simulink model "ZigBee"  (R2017a)
settings: Solver=ode23t  StartTime=0.0  StopTime=inf  FixedStep=SampTime  RelTol=1e-3  EnableMultiTasking=on
PreLoadFcn:
  | %Data Rates
  | BitRate=(250)*1e3;
  | ChipRate=2e6;
  | SymRate=ChipRate/2;
  | OS=32; %Pulse shaping filter oversampling
  | SampRate=OS*SymRate;
  | SampTime=1/SampRate;
  | 
  | %BER overhead
  | RX_ChipDelay=6;
  | 
  | %Signal Specs
  | Pin=-40;
  | fc_RF=2450e6;
  | 
  | %Interference Specs
  | fc_BL=2500e6;
  | INT_CHRT=3.846e6; %chip rate
  | INT_SPS=32; %up-sampling rate
  | INT_RO=0.22; %pulse shaping filter param
  | INT_PWR=0; %passband Power
  | 
  | %Receiver Design + Impairements
  | Gain_LNA=20;
  | IIP2_LNA=inf;
  | IIP3_LNA=inf;
  | NF_LNA=2.5;
  | 
  | Gain_MIX=-5;
  | IIP2_MIX=60;
  | IIP3_MIX=inf;
  | NF_MIX=9;
  | 
  | Gain_VGA=44-15;
  | IIP2_VGA=inf;
  | IIP3_VGA=inf;
  | NF_VGA=12;
  | 
  | ADC_FSP=0;
  | ADC_RES=10;
  | 
  | FLICKER_KERN=2^11;
  | FLICKER_CORNER=10e3;
  | FLICKER_PSD_FLOOR=-124;
  | 
  | PLL_NOISE=[-80 -80 -80 -80 -85 -95];
  | PLL_FREQ=[0.01 0.1 1 2 3 7]*1e6;
  | PLL_KERN=2000;
InitFcn:
  | x=linspace(0,1,OS);
  | weights=sin(pi*x);
undefined symbols (not defined in the file or in its folder): dfilt, Frame, Fs, gcbh, rcfiltgaincompat
libraries: simrfV2elements x9, simulink x5, simrfV2util1 x5, dspstat3 x4, commdigbbndpm3 x3, dspmathops x3, dspobslib x3, simrfV2_lib x3, dspmlti4 x2, dsparch4 x2, commutil2 x1, commrflib2 x1
settings Model: Creator=The MathWorks Inc.  LastModifiedBy=gzucchel
settings DataIOCC: LimitDataPoints=on  SaveFormat=Array  SignalLoggingSaveFormat=ModelDataLogs  SaveOutput=off  SignalLogging=off  DSMLogging=off  SaveTime=off
settings OptimizationCC: ExpressionDepthLimit=2147483647  LifeSpan=inf
settings DebuggingCC: ConsistencyChecking=warning  UnderspecifiedInitializationDetection=Classic  MergeDetectMultiDrivingBlocksExec=none  TimeAdjustmentMsg=warning  MaxConsecutiveZCsMsg=warning  SolverPrmCheckMsg=warning  FcnCallInpInsideContextMsg=warning  ModelReferenceExtraNoncontSigs=warning  StateNameClashWarn=warning  SimStateOlderReleaseMsg=warning  SFUnexpectedBacktrackingDiag=warning  SFNoUnconditionalDefaultTransitionDiag=warning  SFExecutionAtInitializationDiag=none
settings HardwareCC: ProdBitPerPointer=32  ProdBitPerSizeT=32  ProdBitPerPtrDiffT=32  ProdLargestAtomicFloat=None  ProdIntDivRoundTo=Undefined  ProdEndianess=Unspecified  ProdWordSize=32  ProdHWDeviceType=32-bit Generic
settings ModelReferenceCC: PropagateSignalLabelsOutOfModel=off
settings GRTTargetCC: TargetLangStandard=C89/C90 (ANSI)  GeneratePreprocessorConditionals=Disable all  CombineOutputUpdateFcns=off  GRTInterface=on
settings ConfigComp: CovMetricSettings=dw  CovHtmlReporting=on  CovSaveCumulativeToWorkspaceVar=on  CovSaveSingleToWorkspaceVar=on  CovExternalEMLEnable=off  CovSFcnEnable=off
settings ConfigurationSet: Description=SimMechanics 2G

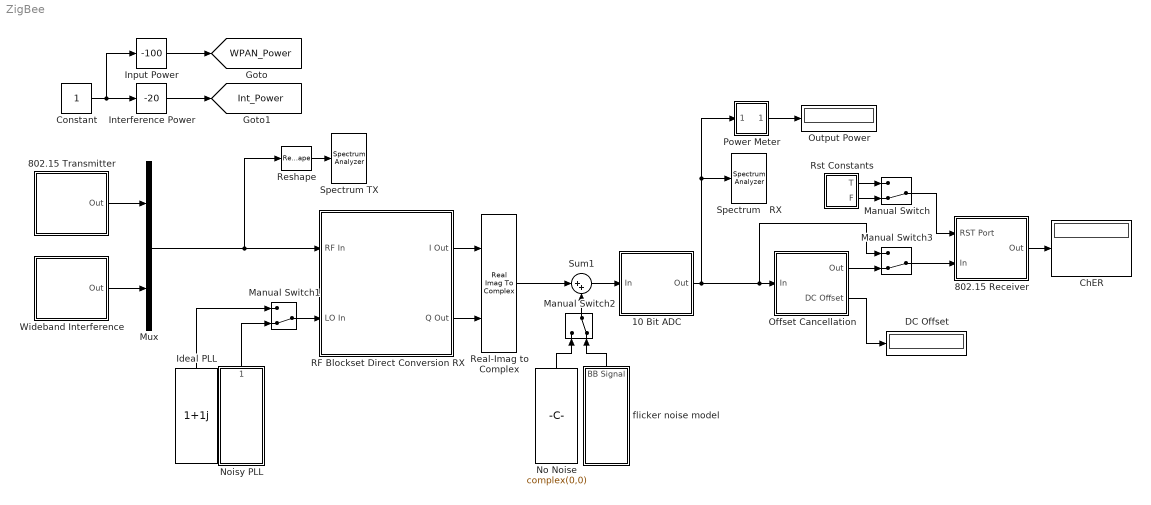
== system ZigBee ==
  10 Bit ADC : Subsystem  mask{FS_P_dBm=0, Rnorm=1, N=10, Sample_Rate=0.0}
      mask prompts: FS_P_dBm "Full Scale Power"; Rnorm "Normalization Resistance"; Sample_Rate "Sample Rate (-1 for inherited)"
      mask init:
      | %LSB=FS_V/(2^(N-1));
      | %MAX=FS_V-LSB;
      | %MIN=-FS_V+LSB;
      | LSB=sqrt(2*Rnorm)*sqrt(1e-3)*sqrt(10^(FS_P_dBm/10))/(2^(N-1));
      | MAXp=sqrt(2*Rnorm)*sqrt(1e-3)*sqrt(10^(FS_P_dBm/10))-LSB;
      | MINp=-sqrt(2*Rnorm)*sqrt(1e-3)*sqrt(10^(FS_P_dBm/10))+LSB;
  802.15 Receiver : Subsystem
  802.15 Transmitter : Subsystem
  ChER : Display
  Constant : Constant
  DC Offset : Display
  Ideal PLL : Constant  Value=1+1j  VectorParams1D=off  SampleTime=1/SampRate  FramePeriod=Frame/Fs
  "Input Power " : simulink/Math Operations/Slider Gain  gain=-100  low=-120  high=-30
  "Interference Power " : simulink/Math Operations/Slider Gain  gain=-20  low=-200  high=0
  Manual Switch{,1..3} (4 alike) : ManualSwitch  CurrentSetting=0
  Mux : Mux  Inputs=2
  No Noise : Constant  Value=complex(0,0)  VectorParams1D=off  SampleTime=1/SampRate  FramePeriod=Frame/Fs
  Noisy PLL : Subsystem  mask{Level_dB=PLL_NOISE, Freq=PLL_FREQ, Fs=SampRate, Npts=PLL_KERN, seed=159775318}
      mask prompts: Level_dB "Noise Level Vector in dBc/Hz"; Freq "Frequency Vector in Hz"; Fs "Sampling Rate in Hz"; Npts "FIR Filter Kernel Length"; seed "Noise Gen Seed"
  Offset Cancellation : Subsystem
  Output Power : Display
  Power Meter : Subsystem  mask{R=1, PB=off, buffer_sz=32*32}
      mask prompts: R "Resistance"; PB "Passband Power (Divide by 2)"; buffer_sz "Buffer Size"
  RF Blockset Direct Conversion RX : Subsystem
  Real-Imag to Complex : RealImagToComplex
  Reshape : Reshape  OutputDimensionality=Row vector (2-D)
  Rst Constants : Subsystem
  Spectrum   RX : SpectrumAnalyzer
  Spectrum TX : SpectrumAnalyzer
  Sum1 : Sum  Inputs=|++
  Wideband Interference : Subsystem
  flicker noise model : Subsystem
  tag scope: Int_Power=global, WPAN_Power=global
  wires:
  802.15 Receiver/1(Out) -> ChER/1
  802.15 Transmitter/1(Out) -> Mux/1
  RF Blockset Direct Conversion RX/1(I Out) -> Real-Imag to Complex/1
  RF Blockset Direct Conversion RX/2(Q Out) -> Real-Imag to Complex/2
  Sum1/1 -> 10 Bit ADC/1(In)
  "Interference Power "/1 -> [Int_Power]
  "Input Power "/1 -> [WPAN_Power]
  10 Bit ADC/1(Out) -> Manual Switch3/1, Offset Cancellation/1(In), Power Meter/1(In), Spectrum   RX/1
  Mux/1 -> RF Blockset Direct Conversion RX/1(RF In), Reshape/1
  Constant/1 -> "Input Power "/1, "Interference Power "/1
  Real-Imag to Complex/1 -> Sum1/1
  Rst Constants/1(T) -> Manual Switch/1
  Rst Constants/2(F) -> Manual Switch/2
  Manual Switch/1 -> 802.15 Receiver/1(RST Port)
  Wideband Interference/1(Out) -> Mux/2
  Manual Switch1/1 -> RF Blockset Direct Conversion RX/2(LO In)
  Noisy PLL/1(PLL Output) -> Manual Switch1/2
  Ideal PLL/1 -> Manual Switch1/1
  Manual Switch2/1 -> Sum1/2
  flicker noise model/1(BB Signal) -> Manual Switch2/2
  No Noise/1 -> Manual Switch2/1
  Power Meter/1(Power) -> Output Power/1
  Offset Cancellation/2(DC Offset) -> DC Offset/1
  Offset Cancellation/1(Out) -> Manual Switch3/2
  Manual Switch3/1 -> 802.15 Receiver/2(In)
  Reshape/1 -> Spectrum TX/1

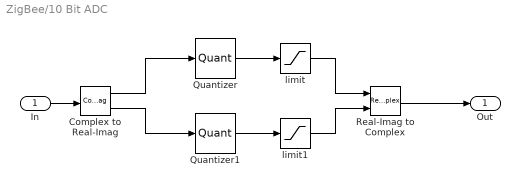
== system ZigBee/10 Bit ADC ==
  In : Inport
  Complex to Real-Imag : ComplexToRealImag
  Quantizer : Quantizer  QuantizationInterval=LSB
  Quantizer1 : Quantizer  QuantizationInterval=LSB
  Real-Imag to Complex : RealImagToComplex
  limit : Saturate  UpperLimit=MAXp  LowerLimit=MINp
  limit1 : Saturate  UpperLimit=MAXp  LowerLimit=MINp
  Out : Outport
  wires:
  Quantizer/1 -> limit/1
  In/1 -> Complex to Real-Imag/1
  Complex to Real-Imag/1 -> Quantizer/1
  Quantizer1/1 -> limit1/1
  Complex to Real-Imag/2 -> Quantizer1/1
  limit/1 -> Real-Imag to Complex/1
  limit1/1 -> Real-Imag to Complex/2
  Real-Imag to Complex/1 -> Out/1

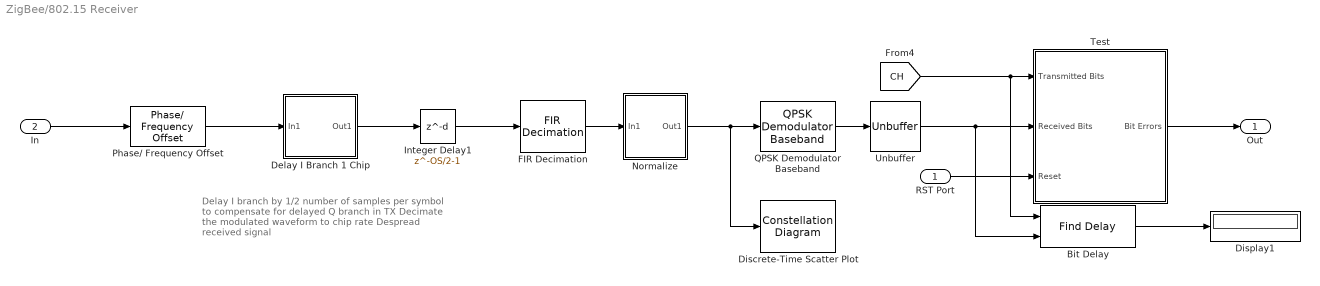
== system ZigBee/802.15 Receiver ==
  note: Delay I branch by 1/2 number of samples per
      | symbol to compensate for delayed Q branch in TX
      |
      | Decimate the modulated waveform to chip rate
      |
      | Despread received signal
  RST Port : Inport
  In : Inport  Port=2
  Bit Delay : commutil2/Find Delay  corrLength=20  chgSigOP=off  stopUpdate=off  numConstDelay=3
      settings: SourceProductName=Communications System Toolbox  SourceProductBaseCode=CM
  Delay I Branch 1 Chip : Subsystem
  Discrete-Time Scatter Plot : ConstellationDiagram  Tag=ScatterPlot
  Display1 : Display
  FIR Decimation : dspmlti4/FIR Decimation  FilterSource=Dialog parameters  h=fliplr(conj(weights))  D=OS  filtStruct=Direct form  FilterObject=Hm_firdecim  InputProcessing=Columns as channels (frame based)  framing=Allow multirate processing  inputOffset=0  outputBufInitCond=0  roundingMode=Floor  overflowMode=off  firstCoeffDataTypeStr=Inherit: Same word length as input  firstCoeffMin=[]  firstCoeffMax=[]  firstCoeffLastDataTypeStr=Inherit: Same word length as input  outputDataTypeStr=Inherit: Same as accumulator  outputMin=[]  outputMax=[]  outputLastDataTypeStr=Inherit: Same as accumulator
  Integer Delay1 : Delay  DelayLength=OS/2-1
  Normalize : Subsystem
  Phase/ Frequency Offset : commrflib2/Phase// Frequency Offset  phaseOffset=58  freqPort=off  freqOffset=0
      settings: SourceProductName=Communications System Toolbox
  QPSK Demodulator Baseband : commdigbbndpm3/QPSK Demodulator Baseband  OutType=Bit  DecType=Hard decision  VarSource=Dialog  Variance=1  Dec=Gray  Ph=pi/4  outDtype1=Inherit via internal rule  outDtype2=Inherit via internal rule  derotateFactorWordLen=16  derotateFactorDataTypeStr=Inherit: Same word length as input  derotateFactorLastDataTypeStr=Inherit: Same word length as input
  Test : Subsystem
  Unbuffer : Unbuffer
  Out : Outport
  wires:
  Test/1(Bit Errors) -> Out/1
  Bit Delay/1 -> Display1/1
  Delay I Branch 1 Chip/1(Out1) -> Integer Delay1/1
  In/1 -> Phase/ Frequency Offset/1
  QPSK Demodulator Baseband/1 -> Unbuffer/1
  Unbuffer/1 -> Test/2(Received Bits), Bit Delay/2
  Integer Delay1/1 -> FIR Decimation/1
  FIR Decimation/1 -> Normalize/1(In1)
  [CH] -> Test/1(Transmitted Bits), Bit Delay/1
  Phase/ Frequency Offset/1 -> Delay I Branch 1 Chip/1(In1)
  Normalize/1(Out1) -> QPSK Demodulator Baseband/1, Discrete-Time Scatter Plot/1
  RST Port/1 -> Test/3(Reset)

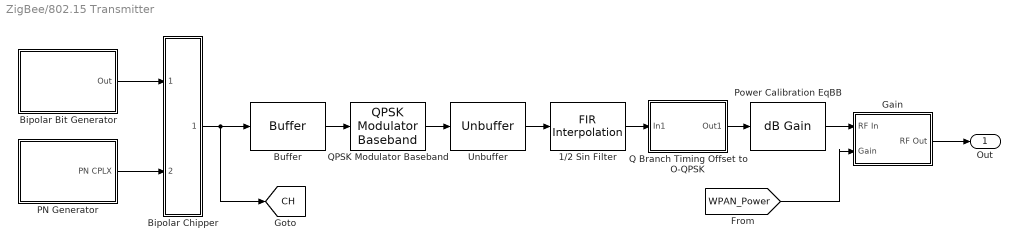
== system ZigBee/802.15 Transmitter ==
  1/2 Sin Filter : dspmlti4/FIR Interpolation  FilterSource=Dialog parameters  h=weights  L=OS  FilterObject=Hm_firinterp  framing=Allow multirate processing  outputBufInitCond=0  roundingMode=Floor  overflowMode=off  firstCoeffDataTypeStr=Inherit: Same word length as input  firstCoeffMin=[]  firstCoeffMax=[]  firstCoeffLastDataTypeStr=Inherit: Same word length as input  outputDataTypeStr=Inherit: Same as accumulator  outputMin=[]  outputMax=[]  outputLastDataTypeStr=Inherit: Same as accumulator
      settings: SourceProductName=DSP System Toolbox
  Bipolar Chipper : Subsystem
  Bipolar Bit Generator : Subsystem
  Buffer : Buffer  N=2
  Gain : Subsystem
  PN Generator : Subsystem
  Power Calibration EqBB : dspmathops/dB Gain  dB=-26.8  intype=Amplitude
      settings: SourceProductName=DSP System Toolbox  SourceProductBaseCode=DS
  Q Branch Timing Offset to O-QPSK : Subsystem
  QPSK Modulator Baseband : commdigbbndpm3/QPSK Modulator Baseband  InType=Bit  Enc=Gray  Ph=pi/4  outDtype=double  outWordLen=16  outUDDataType=sfix(16)  outFracLenMode=Best precision  outFracLen=15  outDataTypeStr=double  outLastDataTypeStr=double
  Unbuffer : Unbuffer
  Out : Outport
  tag scope: CH=global
  wires:
  Power Calibration EqBB/1 -> Gain/1(RF In)
  Gain/1(RF Out) -> Out/1
  Q Branch Timing Offset to O-QPSK/1(Out1) -> Power Calibration EqBB/1
  [WPAN_Power] -> Gain/2(Gain)
  Unbuffer/1 -> 1/2 Sin Filter/1
  Buffer/1 -> QPSK Modulator Baseband/1
  Bipolar Chipper/1(Out) -> [CH], Buffer/1
  Bipolar Bit Generator/1(Out) -> Bipolar Chipper/1(In1)
  PN Generator/1(PN CPLX) -> Bipolar Chipper/2(In2)
  1/2 Sin Filter/1 -> Q Branch Timing Offset to O-QPSK/1(In1)
  QPSK Modulator Baseband/1 -> Unbuffer/1

== system ZigBee/Noisy PLL ==
  Constant : Constant  VectorParams1D=off  SampleTime=1/Fs  FramePeriod=Frame/Fs
  Phase Noise1 : Subsystem  Description=|  mask{Level_dB=Level_dB, Freq=Freq, Fs=Fs, Npts=Npts, seed=seed, Verify=off}
      | User defined phase noise block.
      | Dick Benson, May 2007
      mask prompts: Level_dB "Noise Level Vector in dBc/Hz"; Freq "Frequency Vector in Hz"; Fs "Sampling Rate in Hz"; Npts "FIR Filter Kernel Length (power of 2)"; seed "Noise Gen. Seed"; Verify "Verify Noise Shape Attained"
      mask init:
      | noise_filt=phaseNoise(Npts, Freq, Level_dB, Fs,Verify);
      mask Display: disp('Prototype\nPhase Noise\nBlock')
  Real-Imag to Complex : RealImagToComplex  Input=Real
  PLL Output : Outport
  wires:
  Phase Noise1/1(Out1) -> PLL Output/1
  Real-Imag to Complex/1 -> Phase Noise1/1(In1)
  Constant/1 -> Real-Imag to Complex/1

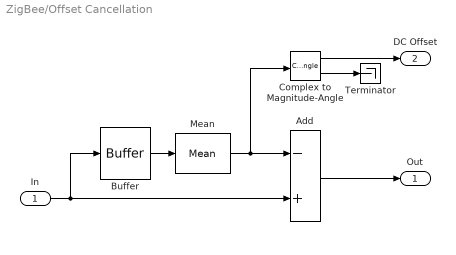
== system ZigBee/Offset Cancellation ==
  In : Inport
  Add : Sum  Inputs=-+
  Buffer : Buffer  N=OS*50  V=OS*25
  Complex to Magnitude-Angle : ComplexToMagnitudeAngle
  Mean : dspstat3/Mean  run=off  reset_popup=None  directionMode=Entire input  dimension=1  roiEnable=off  roiType=Rectangles  roiPortion=Entire ROI  roiOutput=Individual statistics for each ROI  roiFlag=off  outputDataTypeStr=Inherit: Same as accumulator  outputLastDataTypeStr=Inherit: Same as accumulator  outputMin=[]  outputMax=[]  roundingMode=Floor  overflowMode=off
  Terminator : Terminator
  Out : Outport
  DC Offset : Outport  Port=2
  wires:
  Add/1 -> Out/1
  Mean/1 -> Add/1, Complex to Magnitude-Angle/1
  In/1 -> Add/2, Buffer/1
  Buffer/1 -> Mean/1
  Complex to Magnitude-Angle/1 -> DC Offset/1
  Complex to Magnitude-Angle/2 -> Terminator/1

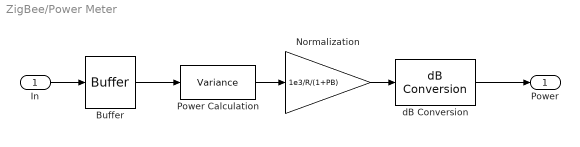
== system ZigBee/Power Meter ==
  In : Inport
  Buffer : Buffer  N=buffer_sz
  Normalization : Gain  Gain=1e3/R/(1+PB)
  Power Calculation : dspstat3/Variance  run=off  reset_popup=None  InputProcessing=Columns as channels (frame based)  directionMode=Each column  dimension=1  roiEnable=off  roiType=Rectangles  roiPortion=Entire ROI  roiOutput=Individual statistics for each ROI  roiFlag=off  roundingMode=Floor  overflowMode=off
      settings: SourceProductName=DSP System Toolbox
  dB Conversion : dspmathops/dB Conversion  dBtype=dB  intype=Power  R=1  fuzz=on
      settings: SourceProductName=DSP System Toolbox
  Power : Outport
  wires:
  Power Calculation/1 -> Normalization/1
  Normalization/1 -> dB Conversion/1
  In/1 -> Buffer/1
  Buffer/1 -> Power Calculation/1
  dB Conversion/1 -> Power/1

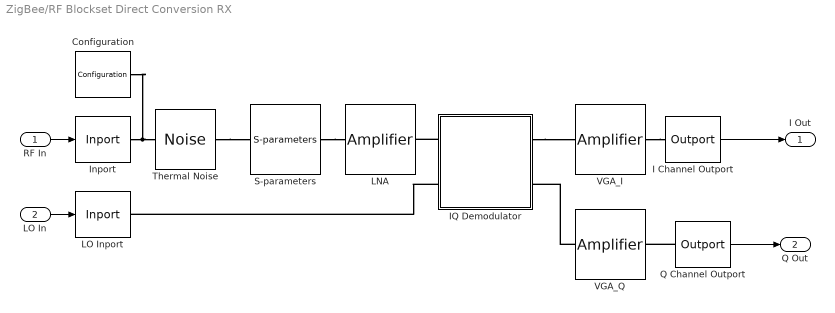
== system ZigBee/RF Blockset Direct Conversion RX ==
  RF In : Inport
  LO In : Inport  Port=2
  Configuration : simrfV2util1/Configuration  AutoFreq=off  Tones="[2.45         2.5] GHz"  Harmonics=[1 3]  NormalizeCarrierPower=on  SolverType=Auto  UseCCode=on  StepSize=SampTime s  AddNoise=on  defaultRNG=on  Seed=0  Temperature=290 K  SolverDelFlag=0  AbsTol=1e-6  RelTol=1e-3  MaxIter=10  ErrorEstimationType=2-norm over all variables
      settings: SourceProductName=RF Blockset  SourceProductBaseCode=RB
  I Channel Outport : simrfV2util1/Outport  SensorType=Power  OutputFormat=Real Passband  CarrierFreq=0 Hz  ZL=100  InternalGrounding=on  StepSize=-1 s  AutoStep=off
      settings: SourceProductName=RF Blockset  SourceProductBaseCode=RB
  IQ Demodulator : Subsystem  DialogController=simrfV2DDGCreate  mask(IQ Demodulator){classname=iqdemod, Source_linear_gain=Available power gain, linear_gain=Gain_MIX, linear_gain_unit=dB, Zin=50, Zout=50, Source_Poly=Even and odd order, Poly_Coeffs=[0 1], IPType=Input, IP2=IIP2_MIX, IP2_unit=dBm, IP3=IIP3_MIX, IP3_unit=dBm, P1dB=inf, P1dB_unit=dBm, Psat=inf, Psat_unit=dBm, Gcomp=inf, Gcomp_unit=dBm, NF=NF_MIX, InternalGrounding=on, LOFreq=0, LOFreq_unit=Hz, GainMismatch=0, GainMismatch_unit=dB, PhaseMismatch=0, PhaseMismatch_unit=deg, Isolation=50, Isolation_unit=dB}
      mask prompts: classname "Class name:"; Source_linear_gain "Gain option:"; linear_gain "Linear gain:"; linear_gain_unit "Linear gain unit:"; Zin "Input impedance:"; Zout "Output impedance:"; Source_Poly "Source of cubic polynomial:"; Poly_Coeffs "Polynomial coefficients:"; IPType "Intercept points at:"; IP2_unit "IP2 unit:"; IP3_unit "IP3 unit:"; P1dB_unit "P1dB unit:"; Psat_unit "Psat unit:"; Gcomp_unit "Gcomp unit:"; NF "Noise figure (dB):"; InternalGrounding "Ground and hide negative terminals."; LOFreq "Local oscillator frequency"; LOFreq_unit "Local oscillator frequency unit:"; GainMismatch "I/Q gain mismatch"; GainMismatch_unit "I/Q gain mismatch unit:"; PhaseMismatch "I/Q phase mismatch:"; PhaseMismatch_unit "I/Q phase mismatch unit:"; Isolation "LO to RF isolation:"; Isolation_unit "LO to RF isolation unit:"
      mask help: Model an IQ demodulator
      mask init:
      | iqDemodMaskParams = simrfV2iqdemod(gcb, 'simrfInit'); % iqDemodMaskParams contains parameters that are verified and converted to standard units
      | 
      | % Assignment to internal block parameters is done only at compile time
      | if regexpi(get_param(bdroot(gcb), 'SimulationStatus'), ...
      |         '^(updating|initializing)$')
      |     % iqDemodParams contains parameters used by internal blocks
      |     iqDemodParams = simrfV2_iqdemod_params(iqDemodMaskParams);
      | end
      mask Help: eval('simrfV2_help(gcbh)')
      mask TypeOptions Source_linear_gain: Available power gain | Open circuit voltage gain | Polynomial coefficients
      mask TypeOptions linear_gain_unit: dB | None
      mask TypeOptions Source_Poly: Even and odd order | Odd order
      mask TypeOptions IPType: Output | Input
      mask TypeOptions IP2_unit: W | mW | dBW | dBm
      mask TypeOptions IP3_unit: W | mW | dBW | dBm
      mask TypeOptions P1dB_unit: W | mW | dBW | dBm
      mask TypeOptions Psat_unit: W | mW | dBW | dBm
      mask TypeOptions Gcomp_unit: W | mW | dBW | dBm
      mask TypeOptions LOFreq_unit: Hz | kHz | MHz | GHz
      mask TypeOptions GainMismatch_unit: dB | None
      mask TypeOptions PhaseMismatch_unit: rad | deg
      mask TypeOptions Isolation_unit: dB | None
      mask Display:
      | simrfV2icon_iqdemod
      | text(0.5+0.15,0.5+0.075,'LO')
      | port_label('LConn', 1,'In')
      | port_label('RConn', 1,'I')
      | port_label('RConn', 2,'Q')
  Inport : simrfV2util1/Inport  SimulinkInputSignalType=Power  CarrierFreq=[fc_RF,fc_BL] Hz  ZS=50  InternalGrounding=on
      settings: SourceProductName=RF Blockset  SourceProductBaseCode=RB
  LNA : simrfV2elements/Amplifier  classname=amplifier  DataSource=Data file  File=unitygain.s2p  Paramtype=S-parameters  Sparam=[0 0;1 0]  SparamFreq=1e9 Hz  SparamZ0=50  Residues=0  Poles=0  DF={0 0; 1 0}  Source_linear_gain=Available power gain  linear_gain=Gain_LNA dB  Zin=50  Zout=50  Source_Poly=Even and odd order  Poly_Coeffs=[0 1]  IPType=Input  IP2=IIP2_LNA dBm  IP3=IIP3_LNA dBm  P1dB=inf dBm  Psat=inf dBm  Gcomp=inf dBm  NF=NF_LNA+1  InternalGrounding=on  SourceFreq=Extracted from data source  PlotFreq=0 Hz  PlotType=X-Y plane  YParam1=S11  YFormat1=Magnitude (decibels)  YParam2=None  YFormat2=Magnitude (decibels)  YOption=Linear  XOption=Linear  SparamRepresentation=Time domain (rationalfit)  FitTol=-40  FitOpt=Fit individually  AutoImpulseLength=off  ImpulseLength=0 s
      settings: SourceProductName=RF Blockset  SourceProductBaseCode=RB
  LO Inport : simrfV2util1/Inport  SimulinkInputSignalType=Ideal voltage  CarrierFreq=fc_RF Hz  ZS=0  InternalGrounding=on
      settings: SourceProductName=RF Blockset  SourceProductBaseCode=RB
  Q Channel Outport : simrfV2util1/Outport  SensorType=Power  OutputFormat=Real Passband  CarrierFreq=0 Hz  ZL=100  InternalGrounding=on  StepSize=-1 s  AutoStep=off
      settings: SourceProductName=RF Blockset  SourceProductBaseCode=RB
  S-parameters : simrfV2elements/S-parameters  classname=sparam_element  DataSource=Data file  File=SAW_Filter_Data.s2p  Paramtype=S-parameters  Sparam=[0 0;1 0]  SparamFreq=1e9 Hz  SparamZ0=50  Residues=0  Poles=0  DF={0 0; 1 0}  FitOpt=Share all poles  FitTol=-40  SourceFreq=Extracted from data source  PlotFreq=1 Hz  PlotType=X-Y plane  YParam1=S21  YFormat1=Magnitude (decibels)  YParam2=None  YFormat2=Magnitude (decibels)  YOption=Linear  XOption=Linear  AddNoise=off  InternalGrounding=on  SparamRepresentation=Time domain (rationalfit)  AutoImpulseLength=off  ImpulseLength=0 s
      settings: SourceProductName=RF Blockset  SourceProductBaseCode=RB
  Thermal Noise : simrfV2sources1/Noise  SimulinkInputSignalType=Ideal voltage  NoiseType=White  NoisePSD=4*1.381e-23*290*50  CarrierFreq=fc_RF Hz  InternalGrounding=off
      settings: SourceProductName=RF Blockset  SourceProductBaseCode=RB
  VGA_I : simrfV2elements/Amplifier  classname=amplifier  DataSource=Data file  File=unitygain.s2p  Paramtype=S-parameters  Sparam=[0 0;1 0]  SparamFreq=1e9 Hz  SparamZ0=50  Residues=0  Poles=0  DF={0 0; 1 0}  Source_linear_gain=Available power gain  linear_gain=Gain_VGA dB  Zin=100  Zout=100  Source_Poly=Even and odd order  Poly_Coeffs=[0 1]  IPType=Input  IP2=IIP2_VGA dBm  IP3=IIP3_VGA dBm  P1dB=inf dBm  Psat=inf dBm  Gcomp=inf dBm  NF=NF_VGA  InternalGrounding=on  SourceFreq=Extracted from data source  PlotFreq=0 Hz  PlotType=X-Y plane  YParam1=S11  YFormat1=Magnitude (decibels)  YParam2=None  YFormat2=Magnitude (decibels)  YOption=Linear  XOption=Linear  SparamRepresentation=Time domain (rationalfit)  FitTol=-40  FitOpt=Fit individually  AutoImpulseLength=off  ImpulseLength=0 s
      settings: SourceProductName=RF Blockset  SourceProductBaseCode=RB
  VGA_Q : simrfV2elements/Amplifier  classname=amplifier  DataSource=Data file  File=unitygain.s2p  Paramtype=S-parameters  Sparam=[0 0;1 0]  SparamFreq=1e9 Hz  SparamZ0=50  Residues=0  Poles=0  DF={0 0; 1 0}  Source_linear_gain=Available power gain  linear_gain=Gain_VGA dB  Zin=100  Zout=100  Source_Poly=Even and odd order  Poly_Coeffs=[0 1]  IPType=Input  IP2=IIP2_VGA dBm  IP3=IIP3_VGA dBm  P1dB=inf dBm  Psat=inf dBm  Gcomp=inf dBm  NF=NF_VGA  InternalGrounding=on  SourceFreq=Extracted from data source  PlotFreq=0 Hz  PlotType=X-Y plane  YParam1=S11  YFormat1=Magnitude (decibels)  YParam2=None  YFormat2=Magnitude (decibels)  YOption=Linear  XOption=Linear  SparamRepresentation=Time domain (rationalfit)  FitTol=-40  FitOpt=Fit individually  AutoImpulseLength=off  ImpulseLength=0 s
      settings: SourceProductName=RF Blockset  SourceProductBaseCode=RB
  I Out : Outport
  Q Out : Outport  Port=2
  wires:
  LO In/1 -> LO Inport/1
  RF In/1 -> Inport/1
  Q Channel Outport/1 -> Q Out/1
  I Channel Outport/1 -> I Out/1
  connections:
  VGA_I/RConn1 -- I Channel Outport/LConn1
  Q Channel Outport/LConn1 -- VGA_Q/RConn1
  VGA_Q/LConn1 -- IQ Demodulator/RConn2
  IQ Demodulator/RConn1 -- VGA_I/LConn1
  Inport/RConn1 -- Configuration/LConn1 -- Thermal Noise/RConn1
  S-parameters/RConn1 -- LNA/LConn1
  Thermal Noise/LConn1 -- S-parameters/LConn1
  IQ Demodulator/LConn1 -- LNA/RConn1
  IQ Demodulator/LConn2 -- LO Inport/RConn1

== system ZigBee/Rst Constants ==
  Constant : Constant
  Constant1 : Constant  Value=0
  T : Outport
  F : Outport  Port=2
  wires:
  Constant/1 -> T/1
  Constant1/1 -> F/1

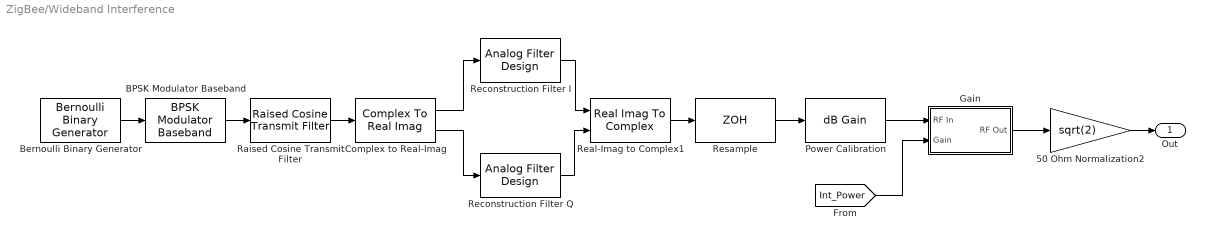
== system ZigBee/Wideband Interference ==
  50 Ohm Normalization2 : Gain  Gain=sqrt(2)
  BPSK Modulator Baseband : commdigbbndpm3/BPSK Modulator Baseband  Ph=0  outDtype=double  outWordLen=16  outUDDataType=sfix(16)  outFracLenMode=Best precision  outFracLen=15  outDataTypeStr=double  outLastDataTypeStr=double
  Bernoulli Binary Generator : commrandsrc2/Bernoulli Binary Generator  P=0.5  seed=61  Ts=1/INT_CHRT  frameBased=off  sampPerFrame=1  orient=off  outDataType=double
  Complex to Real-Imag : ComplexToRealImag
  Gain : Subsystem
  Power Calibration : dspmathops/dB Gain  dB=-17.95  intype=Amplitude
      settings: SourceProductName=DSP System Toolbox  SourceProductBaseCode=DS
  Raised Cosine Transmit Filter : commfilt2/Raised Cosine Transmit Filter  filtType=Square root  R=INT_RO  filtSpan=2*(6)  N=INT_SPS  filterGain=rcfiltgaincompat(gcbh)  RateOptions=Allow multirate processing  framing=Mute  checkCoeff=off  variableName=rcTxFilt  checkGain=Normalized  sampMode=Mute  saveAsFlag=0  currentFiltSpan=2*(6)  D=6  launchFVT=off  roundingMode=Floor  overflowMode=off  coeffDataTypeStr=Inherit: Same word length as input  coeffMin=[]  coeffMax=[]  coeffLastDataTypeStr=Inherit: Same word length as input  outputDataTypeStr=Inherit: Same as accumulator  outputMin=[]  outputMax=[]  outputLastDataTypeStr=Inherit: Same as accumulator
  Real-Imag to Complex1 : RealImagToComplex
  Reconstruction Filter I : dsparch4/Analog Filter Design  method=Butterworth  filttype=Lowpass  N=8  Wlo=2*pi/SampTime  Whi=80  Rp=2  Rs=40
  Reconstruction Filter Q : dsparch4/Analog Filter Design  method=Butterworth  filttype=Lowpass  N=8  Wlo=2*pi/SampTime  Whi=80  Rp=2  Rs=40
  Resample : ZeroOrderHold  SampleTime=SampTime
  Out : Outport
  wires:
  [Int_Power] -> Gain/2(Gain)
  Power Calibration/1 -> Gain/1(RF In)
  Resample/1 -> Power Calibration/1
  BPSK Modulator Baseband/1 -> Raised Cosine Transmit Filter/1
  Bernoulli Binary Generator/1 -> BPSK Modulator Baseband/1
  Raised Cosine Transmit Filter/1 -> Complex to Real-Imag/1
  Complex to Real-Imag/2 -> Reconstruction Filter Q/1
  Complex to Real-Imag/1 -> Reconstruction Filter I/1
  Real-Imag to Complex1/1 -> Resample/1
  Reconstruction Filter I/1 -> Real-Imag to Complex1/1
  Reconstruction Filter Q/1 -> Real-Imag to Complex1/2
  Gain/1(RF Out) -> 50 Ohm Normalization2/1
  50 Ohm Normalization2/1 -> Out/1

== system ZigBee/flicker noise model ==
  I Channel Flicker Noise : Subsystem  mask{Npts=FLICKER_KERN, Fs=SymRate*OS, fcorner=FLICKER_CORNER, Pcorner_dBm=FLICKER_PSD_FLOOR, R=1, seed=12345}
      mask prompts: Npts "Filter Kernel Size"; Fs "Sampling Frequency (Hz)"; fcorner "Flicker Noise Corner Frequency (Hz)"; Pcorner_dBm "Single Sided System Noise Floor (dBm/Hz)"; R "Reference Impedance"; seed "Random Seed"
      mask init:
      | noise_filt=pinkNoise(Npts, Fs, fcorner, Pcorner_dBm,R);
  Q Channel Flicker Noise : Subsystem  mask{Npts=FLICKER_KERN, Fs=SymRate*OS, fcorner=FLICKER_CORNER, Pcorner_dBm=FLICKER_PSD_FLOOR, R=1, seed=67543}
      mask prompts: Npts "Filter Kernel Size"; Fs "Sampling Frequency (Hz)"; fcorner "Flicker Noise Corner Frequency (Hz)"; Pcorner_dBm "Single Sided System Noise Floor (dBm/Hz)"; R "Reference Impedance"; seed "Random Seed"
      mask init:
      | noise_filt=pinkNoise(Npts, Fs, fcorner, Pcorner_dBm,R);
  Real-Imag to Complex1 : RealImagToComplex
  BB Signal : Outport
  wires:
  I Channel Flicker Noise/1(Baseband Noise) -> Real-Imag to Complex1/1
  Q Channel Flicker Noise/1(Baseband Noise) -> Real-Imag to Complex1/2
  Real-Imag to Complex1/1 -> BB Signal/1

== system ZigBee/802.15 Receiver/Delay I Branch 1 Chip ==
  In1 : Inport
  Complex to Real-Imag : ComplexToRealImag
  Integer Delay : Delay  DelayLength=OS/2
  Real-Imag to Complex : RealImagToComplex
  Out1 : Outport
  wires:
  Complex to Real-Imag/1 -> Integer Delay/1
  Integer Delay/1 -> Real-Imag to Complex/1
  Complex to Real-Imag/2 -> Real-Imag to Complex/2
  In1/1 -> Complex to Real-Imag/1
  Real-Imag to Complex/1 -> Out1/1

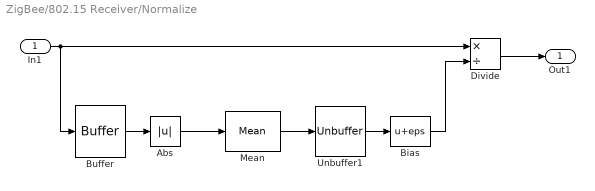
== system ZigBee/802.15 Receiver/Normalize ==
  In1 : Inport
  Abs : Abs
  Bias : Bias  Bias=eps
  Buffer : Buffer
  Divide : Product  Inputs=*/
  Mean : dspstat3/Mean  run=off  reset_popup=None  InputProcessing=Columns as channels (frame based)  directionMode=Each column  dimension=1  roiEnable=off  roiType=Rectangles  roiPortion=Entire ROI  roiOutput=Individual statistics for each ROI  roiFlag=off  outputDataTypeStr=Inherit: Same as accumulator  outputLastDataTypeStr=Inherit: Same as accumulator  outputMin=[]  outputMax=[]  roundingMode=Floor  overflowMode=off
  Unbuffer1 : Unbuffer
  Out1 : Outport
  wires:
  Buffer/1 -> Abs/1
  Abs/1 -> Mean/1
  Mean/1 -> Unbuffer1/1
  In1/1 -> Buffer/1, Divide/1
  Divide/1 -> Out1/1
  Unbuffer1/1 -> Bias/1
  Bias/1 -> Divide/2

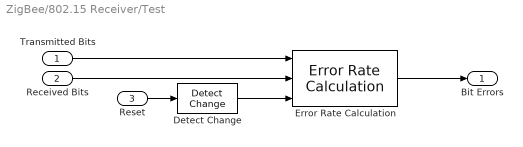
== system ZigBee/802.15 Receiver/Test ==
  Transmitted Bits : Inport
  Received Bits : Inport  Port=2
  Reset : Inport  Port=3
  Detect Change : simulink/Logic and Bit Operations/Detect Change  vinit=1  OutDataTypeStr=boolean
  Error Rate Calculation : commsink2/Error Rate Calculation  N=6  st_delay=200 %additional delay for DC offset correction  cp_mode=Entire frame  subframe=[]  PMode=Port  WsName=ErrorVec  RsMode2=on  stop=off  numErr=inf  maxBits=1000
  Bit Errors : Outport
  wires:
  Transmitted Bits/1 -> Error Rate Calculation/1
  Error Rate Calculation/1 -> Bit Errors/1
  Received Bits/1 -> Error Rate Calculation/2
  Reset/1 -> Detect Change/1
  Detect Change/1 -> Error Rate Calculation/3

== system ZigBee/802.15 Transmitter/Bipolar Chipper ==
  In1 : Inport
  In2 : Inport  Port=2
  Level Shifter : Subsystem
  Product : Product  RndMeth=Zero
  Out : Outport
  wires:
  Product/1 -> Level Shifter/1(In)
  In1/1 -> Product/1
  Level Shifter/1(Out) -> Out/1
  In2/1 -> Product/2

== system ZigBee/802.15 Transmitter/Bipolar Bit Generator ==
  Bernoulli Binary Generator : commrandsrc3/Bernoulli Binary Generator  ProbabilityOfZero=0.5  SeedSource=Parameter  Seed=61  SampleTime=1/BitRate  SamplesPerFrame=1  OutputDataType=double  SimulateUsing=Interpreted execution
  Level Shifter : Subsystem
  Out : Outport
  wires:
  Bernoulli Binary Generator/1 -> Level Shifter/1(In)
  Level Shifter/1(Out) -> Out/1

== system ZigBee/802.15 Transmitter/Gain ==
  RF In : Inport
  Gain : Inport  Port=2
  Gain X : Gain  Gain=1/20
  Math Function : Math  Operator=10^u  SaturateOnIntegerOverflow=on
  Product : Product  RndMeth=Zero
  RF Out : Outport
  wires:
  Gain X/1 -> Math Function/1
  Math Function/1 -> Product/2
  RF In/1 -> Product/1
  Product/1 -> RF Out/1
  Gain/1 -> Gain X/1

== system ZigBee/802.15 Transmitter/PN Generator ==
  Level Shifter : Subsystem
  Scrambling code : commseqgen2/PN Sequence Generator  poly=[0 -7 -10]  ini_sta=[1 0 0 0 0 0 0 0 0 0]  outBitMaskSource=Dialog parameter  shift=0  outVarSiz=off  maxOutSizeMode=Dialog parameter  maxOutSize=[10 1]  Ts=1/ChipRate  frameBased=off  sampPerFrame=1  reset=off  bitPackedOutputs=off  outDataType=double  numPackedBits=8  bitPackDataSigned=off  bitPackedOutDType=double
  PN CPLX : Outport
  wires:
  Scrambling code/1 -> Level Shifter/1(In)
  Level Shifter/1(Out) -> PN CPLX/1

== system ZigBee/802.15 Transmitter/Q Branch Timing Offset to O-QPSK ==
  In1 : Inport
  Complex to Real-Imag : ComplexToRealImag
  Integer Delay : Delay  DelayLength=OS/2
  Real-Imag to Complex : RealImagToComplex
  Out1 : Outport
  wires:
  Complex to Real-Imag/2 -> Integer Delay/1
  Integer Delay/1 -> Real-Imag to Complex/2
  Complex to Real-Imag/1 -> Real-Imag to Complex/1
  In1/1 -> Complex to Real-Imag/1
  Real-Imag to Complex/1 -> Out1/1

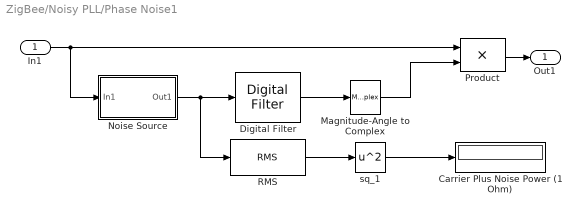
== system ZigBee/Noisy PLL/Phase Noise1 ==
  In1 : Inport
  Carrier Plus Noise Power (1 Ohm) : Display
  Digital Filter : dspobslib/Digital Filter  TypePopup=FIR (all zeros)  IIRFiltStruct=Direct form II transposed  AllPoleFiltStruct=Direct form  FIRFiltStruct=Direct form  CoeffSource=Specify via dialog  NumCoeffs=noise_filt*sqrt(Fs)  DenCoeffs=den  BiQuadCoeffs=[1 0.3 0.4 1 0.1 0.2]  LatticeCoeffs=[0.2 0.4]  denIgnore=on  FiltPerSampPopup=One filter per frame  IC=0  ICnum=0  ICden=0  roundingMode=Floor  overflowMode=off  ScaleValues=1  scaleValueFracLength=14  stageInFracLength=15  stageOutFracLength=15  FilterSource=Specify via dialog  dfiltObjectName=dfilt.dffir([1 2 1])  InputProcessing=Inherited (this choice will be removed - see release notes)
      settings: SourceProductName=DSP System Toolbox  SourceProductBaseCode=DS
  Magnitude-Angle to Complex : MagnitudeAngleToComplex  Input=Angle  ConstantPart=1
  Noise Source : Subsystem
      mask Display: disp('Noise Source')
  Product : Product  SaturateOnIntegerOverflow=on  InputSameDT=on  OutDataTypeStr=Inherit: Same as first input
  RMS : dspstat3/RMS  run=off  directionMode=Each column  dimension=1  InputProcessing=Columns as channels (frame based)  reset_popup=None
  sq_1 : Math  Operator=square  SaturateOnIntegerOverflow=on
  Out1 : Outport
  wires:
  Magnitude-Angle to Complex/1 -> Product/2
  Noise Source/1(Out1) -> Digital Filter/1, RMS/1
  Digital Filter/1 -> Magnitude-Angle to Complex/1
  In1/1 -> Noise Source/1(In1), Product/1
  Product/1 -> Out1/1
  sq_1/1 -> Carrier Plus Noise Power (1 Ohm)/1
  RMS/1 -> sq_1/1

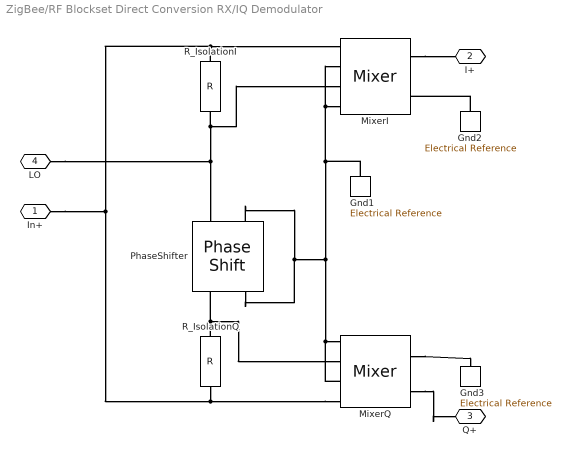
== system ZigBee/RF Blockset Direct Conversion RX/IQ Demodulator ==
  Gnd1 : simrfV2_lib/Elements/Electrical Reference
  Gnd2 : simrfV2_lib/Elements/Electrical Reference
  Gnd3 : simrfV2_lib/Elements/Electrical Reference
  MixerI : simrfV2elements/Mixer  classname=mixer  Source_linear_gain=Available power gain  linear_gain=iqDemodParams.MixerI.Gain dB  Zin=iqDemodParams.MixerI.Zin  Zout=iqDemodParams.MixerI.Zout  ZLO=inf  Source_Poly=Even and odd order  Poly_Coeffs=iqDemodParams.MixerI.Poly_Coeffs  IPType=Input  IP2=iqDemodParams.MixerI.IP2 dBm  IP3=iqDemodParams.MixerI.IP3 dBm  P1dB=iqDemodParams.MixerI.P1dB dBm  Psat=iqDemodParams.MixerI.Psat dBm  Gcomp=iqDemodParams.MixerI.Gcomp dBm  NF=iqDemodParams.MixerI.NF  InternalGrounding=off
      settings: SourceProductName=SimRF  SourceProductBaseCode=RB
  MixerQ : simrfV2elements/Mixer  classname=mixer  Source_linear_gain=Available power gain  linear_gain=iqDemodParams.MixerQ.Gain dB  Zin=iqDemodParams.MixerQ.Zin  Zout=iqDemodParams.MixerQ.Zout  ZLO=inf  Source_Poly=Even and odd order  Poly_Coeffs=iqDemodParams.MixerQ.Poly_Coeffs  IPType=Input  IP2=iqDemodParams.MixerQ.IP2 dBm  IP3=iqDemodParams.MixerQ.IP3 dBm  P1dB=iqDemodParams.MixerQ.P1dB dBm  Psat=iqDemodParams.MixerQ.Psat dBm  Gcomp=iqDemodParams.MixerQ.Gcomp dBm  NF=iqDemodParams.MixerQ.NF  InternalGrounding=off
      settings: SourceProductName=SimRF  SourceProductBaseCode=RB
  PhaseShifter : simrfV2elements/Phase Shift  PhaseShift=iqDemodParams.PhaseShifter.PhaseShift deg  InternalGrounding=off
      settings: SourceProductName=SimRF  SourceProductBaseCode=RB
  R_IsolationI : simrfV2elements/R  classname=resistor  Resistance=iqDemodParams.R_IsolationI.Resistance Ohm  AddNoise=off
      settings: SourceProductName=SimRF  SourceProductBaseCode=RB
  R_IsolationQ : simrfV2elements/R  classname=resistor  Resistance=iqDemodParams.R_IsolationQ.Resistance Ohm  AddNoise=off
      settings: SourceProductName=SimRF  SourceProductBaseCode=RB
  In+ : PMIOPort  Port=1  Side=Left
  I+ : PMIOPort  Port=2  Side=Right
  Q+ : PMIOPort  Port=3  Side=Right
  LO : PMIOPort  Port=4  Side=Left
  connections:
  MixerI/RConn1 -- I+/RConn1
  Gnd2/LConn1 -- MixerI/RConn2
  MixerQ/RConn1 -- Q+/RConn1
  MixerQ/RConn2 -- Gnd3/LConn1
  MixerI/LConn4 -- MixerI/LConn2 -- Gnd1/LConn1 -- MixerQ/LConn4 -- MixerQ/LConn2 -- PhaseShifter/RConn2 -- PhaseShifter/LConn2
  PhaseShifter/RConn1 -- R_IsolationQ/RConn1 -- MixerQ/LConn3
  R_IsolationI/RConn1 -- MixerI/LConn3 -- LO/RConn1 -- PhaseShifter/LConn1
  MixerQ/LConn1 -- R_IsolationQ/LConn1 -- In+/RConn1 -- R_IsolationI/LConn1 -- MixerI/LConn1

== system ZigBee/Wideband Interference/Gain ==
  RF In : Inport
  Gain : Inport  Port=2
  Gain X : Gain  Gain=1/20
  Math Function : Math  Operator=10^u  SaturateOnIntegerOverflow=on
  Product : Product  RndMeth=Zero
  RF Out : Outport
  wires:
  Gain/1 -> Gain X/1
  Product/1 -> RF Out/1
  RF In/1 -> Product/1
  Math Function/1 -> Product/2
  Gain X/1 -> Math Function/1

== system ZigBee/flicker noise model/I Channel Flicker Noise ==
  Band-Limited White Noise : simulink/Sources/Band-Limited White Noise  Cov=1  Ts=1/Fs  seed=seed
  Digital Filter : dspobslib/Digital Filter  TypePopup=FIR (all zeros)  IIRFiltStruct=Direct form II  AllPoleFiltStruct=Direct form  FIRFiltStruct=Direct form  CoeffSource=Specify via dialog  NumCoeffs=noise_filt  DenCoeffs=a  BiQuadCoeffs=[1 0.3 0.4 1 0.1 0.2]  LatticeCoeffs=[0.2 0.4]  denIgnore=on  FiltPerSampPopup=One filter per frame  IC=0  ICnum=0  ICden=0  roundingMode=Floor  overflowMode=off  ScaleValues=1  scaleValueFracLength=14  stageInFracLength=15  stageOutFracLength=15  FilterSource=Specify via dialog  dfiltObjectName=dfilt.dffir([1 2 1])
      settings: SourceProductName=DSP System Toolbox  SourceProductBaseCode=DS
  Baseband Noise : Outport
  wires:
  Band-Limited White Noise/1 -> Digital Filter/1
  Digital Filter/1 -> Baseband Noise/1

== system ZigBee/flicker noise model/Q Channel Flicker Noise ==
  Band-Limited White Noise : simulink/Sources/Band-Limited White Noise  Cov=1  Ts=1/Fs  seed=seed
  Digital Filter : dspobslib/Digital Filter  TypePopup=FIR (all zeros)  IIRFiltStruct=Direct form II  AllPoleFiltStruct=Direct form  FIRFiltStruct=Direct form  CoeffSource=Specify via dialog  NumCoeffs=noise_filt  DenCoeffs=a  BiQuadCoeffs=[1 0.3 0.4 1 0.1 0.2]  LatticeCoeffs=[0.2 0.4]  denIgnore=on  FiltPerSampPopup=One filter per frame  IC=0  ICnum=0  ICden=0  roundingMode=Floor  overflowMode=off  ScaleValues=1  scaleValueFracLength=14  stageInFracLength=15  stageOutFracLength=15  FilterSource=Specify via dialog  dfiltObjectName=dfilt.dffir([1 2 1])
      settings: SourceProductName=DSP System Toolbox  SourceProductBaseCode=DS
  Baseband Noise : Outport
  wires:
  Digital Filter/1 -> Baseband Noise/1
  Band-Limited White Noise/1 -> Digital Filter/1

== system ZigBee/802.15 Transmitter/Bipolar Chipper/Level Shifter ==
  In : Inport
  Bias : Bias  Bias=1
  Gain : Gain  Gain=0.5
  Out : Outport
  wires:
  Bias/1 -> Gain/1
  In/1 -> Bias/1
  Gain/1 -> Out/1

== system ZigBee/802.15 Transmitter/Bipolar Bit Generator/Level Shifter ==
  In : Inport
  Bias : Bias  Bias=-1
  Gain : Gain  Gain=2
  Out : Outport
  wires:
  Gain/1 -> Bias/1
  In/1 -> Gain/1
  Bias/1 -> Out/1

== system ZigBee/802.15 Transmitter/PN Generator/Level Shifter ==
  In : Inport
  Bias : Bias  Bias=-1
  Gain : Gain  Gain=2
  Out : Outport
  wires:
  Gain/1 -> Bias/1
  Bias/1 -> Out/1
  In/1 -> Gain/1

== system ZigBee/Noisy PLL/Phase Noise1/Noise Source ==
  In1 : Inport
  AWGN Channel : commchan3/AWGN Channel  InputProcessing=Inherited (this choice will be removed - see release notes)  seed=12598763  noiseMode=Variance from mask  EbNodB=10  EsNodB=10  SNRdB=0  bitsPerSym=1  Ps=1  Tsym=1  variance=2
  Complex to Real-Imag : ComplexToRealImag  Output=Real
  Sum : Sum  Inputs=-+|  SaturateOnIntegerOverflow=on  InputSameDT=on  OutDataTypeStr=Inherit: Same as first input
  Out1 : Outport
  wires:
  Complex to Real-Imag/1 -> Out1/1
  In1/1 -> Sum/1, AWGN Channel/1
  AWGN Channel/1 -> Sum/2
  Sum/1 -> Complex to Real-Imag/1
